simulink model "f_trigger_queuetest"  (R2018a)
settings: Solver=VariableStepAuto  StartTime=0.0  StopTime=10  RelTol=1e-3
libraries: dspsigops x2, dspbuff3 x1
settings Model: Creator=Michael Girbino  LastModifiedBy=Michael Girbino

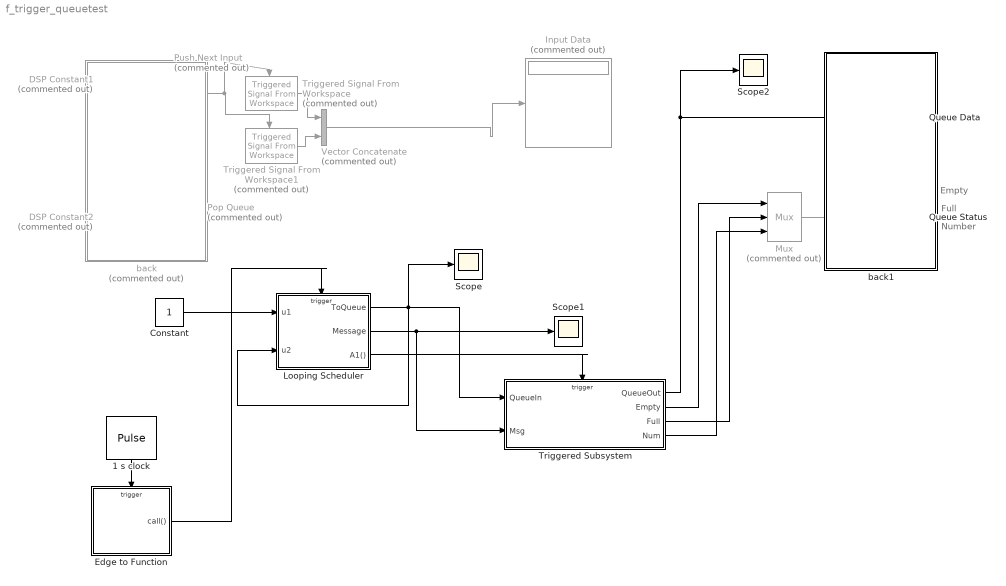
== system f_trigger_queuetest ==
  note: Empty
  note: Full
  note: Number
  1 s clock : DiscretePulseGenerator  PulseType=Time based  Period=1  PulseWidth=10
  Constant : Constant
  DSP Constant1 : Constant  Commented=on  SampleTime=4
  DSP Constant2 : Constant  Commented=on  Value=0  SampleTime=4
  "Edge to Function " : Stateflow chart  TreatAsAtomicUnit=on
  Input Data : Display  Commented=on
  Looping Scheduler : Stateflow chart  TreatAsAtomicUnit=on
  Mux : Mux  Commented=on  Inputs=3
      settings: DisplayOption=signals
  Pop Queue : ManualSwitch  Commented=on
  Push Next Input : ManualSwitch  Commented=on  CurrentSetting=0
  Queue Data : Display
  Queue Status : Display
  Scope : Scope
  Scope1 : Scope
  Scope2 : Scope
  Triggered Subsystem : Subsystem  TreatAsAtomicUnit=on
  Triggered Signal From Workspace : dspsigops/Triggered Signal From Workspace  Commented=on  Signal=1:32  TriggerType=Either edge  ic=0  SamplesPerFrame=1  OutputAfterFinalValue=Setting to zero  OutputFrames=off
      settings: SourceProductName=DSP System Toolbox  SourceProductBaseCode=DS
  Triggered Signal From Workspace1 : dspsigops/Triggered Signal From Workspace  Commented=on  Signal=4:36  TriggerType=Either edge  ic=0  SamplesPerFrame=1  OutputAfterFinalValue=Setting to zero  OutputFrames=off
      settings: SourceProductName=DSP System Toolbox  SourceProductBaseCode=DS
  Vector Concatenate : Concatenate  Commented=on
  back : Subsystem  Commented=on
  back1 : Subsystem
  wires:
  Triggered Signal From Workspace1/1 -> Vector Concatenate/2
  Triggered Signal From Workspace/1 -> Vector Concatenate/1
  DSP Constant1/1 -> Pop Queue/1, Push Next Input/1
  DSP Constant2/1 -> Pop Queue/2, Push Next Input/2
  Push Next Input/1 -> Triggered Signal From Workspace1/Trigger, Triggered Signal From Workspace/Trigger
  Vector Concatenate/1 -> Input Data/1
  Mux/1 -> Queue Status/1
  Triggered Subsystem/1(QueueOut) -> Scope2/1, Queue Data/1
  Triggered Subsystem/2(Empty) -> Mux/1
  Triggered Subsystem/3(Full) -> Mux/2
  Triggered Subsystem/4(Num) -> Mux/3
  Looping Scheduler/3(A1()) -> Triggered Subsystem/Trigger
  Looping Scheduler/1(ToQueue) -> Looping Scheduler/2(u2), Scope/1, Triggered Subsystem/1(QueueIn)
  Looping Scheduler/2(Message) -> Scope1/1, Triggered Subsystem/2(Msg)
  1 s clock/1 -> "Edge to Function "/Trigger
  "Edge to Function "/1(call()) -> Looping Scheduler/Trigger
  Constant/1 -> Looping Scheduler/1(u1)

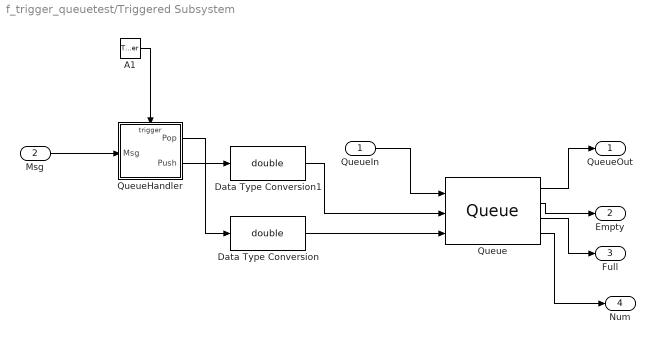
== system f_trigger_queuetest/Triggered Subsystem ==
  QueueIn : Inport  OutDataTypeStr=double
  Msg : Inport  Port=2  OutDataTypeStr=double
  A1 : TriggerPort  TriggerType=function-call  VariantControl=Variant  ShowOutputPort=on  OutputDataType=int8  PortDimensions=1
  Data Type Conversion : DataTypeConversion  OutDataTypeStr=double
  Data Type Conversion1 : DataTypeConversion  OutDataTypeStr=double
  Queue : dspbuff3/Queue  depth=8  trigger=Either edge  overflow=Dynamic reallocation  pes=Warning  eso=on  fso=on  nso=on  clr=off  clrOutport=off  adf=on
      settings: SourceProductName=DSP System Toolbox  SourceProductBaseCode=DS
  QueueHandler : Stateflow chart  TreatAsAtomicUnit=on
  QueueOut : Outport  OutDataTypeStr=double
  Empty : Outport  Port=2  OutDataTypeStr=boolean
  Full : Outport  Port=3  OutDataTypeStr=boolean
  Num : Outport  Port=4  OutDataTypeStr=double
  wires:
  QueueIn/1 -> Queue/1
  Queue/1 -> QueueOut/1
  Queue/2 -> Empty/1
  Queue/3 -> Full/1
  Queue/4 -> Num/1
  QueueHandler/1(Pop) -> Data Type Conversion/1
  Data Type Conversion/1 -> Queue/3
  Msg/1 -> QueueHandler/1(Msg)
  A1/1 -> QueueHandler/Trigger
  QueueHandler/2(Push) -> Data Type Conversion1/1
  Data Type Conversion1/1 -> Queue/2

== system f_trigger_queuetest/back ==

== system f_trigger_queuetest/back1 ==

== stateflow chart f_trigger_queuetest/Looping Scheduler ==
  (default) -> (junction 5) : {ToQueue=1;}
  (junction 6) -> (junction 5) [order 1] : [ToQueue<=8]
      | {
      | %ToQueue = i;
      | Message = 1;
      | send(A1);
      | ToQueue = u1+u2;
      | }
  (junction 5) -> (junction 6)
  (junction 6) -> (junction 20) [order 2] : {i=1;}
  (junction 17) -> (junction 20) [commented out] : [i<=8]
      | {
      | Message = 2;
      | send(A1);
      | i = i + 1;
      | }
  (junction 20) -> (junction 17) [commented out]
  (junction 17) -> (junction 23) [commented out]
  data: i local double; ToQueue output double; Message output double; u1 input double; u2 input double
  events: A1 output FUNCTION_CALL_EVENT; call input FUNCTION_CALL_EVENT

== stateflow chart f_trigger_queuetest/Edge to Function  ==
  (default) -> (junction 2) : {call;}
  events: edge input RISING_EDGE_EVENT; call output FUNCTION_CALL_EVENT

== stateflow chart f_trigger_queuetest/Triggered Subsystem/QueueHandler ==
  (default) -> (junction 19)
  (junction 19) -> (junction 20) [order 1] : [Msg == 1]
  (junction 19) -> (junction 21) [order 2]
  (junction 20) -> (junction 25) : {send(Push);}
  (junction 21) -> (junction 22) [order 1] : [Msg == 2]
  (junction 21) -> (junction 23) [order 2]
  (junction 22) -> (junction 24) : {send(Pop);}
  (junction 24) -> (junction 23)
  (junction 25) -> (junction 24)
  (junction 23) -> (junction 26)
  data: Msg input double
  events: Pop output EITHER_EDGE_EVENT; Push output EITHER_EDGE_EVENT; Run input EITHER_EDGE_EVENT
